simulink model "ModelloParametroNonNoto"  (R2025b)
settings: Solver=ode45  StartTime=0.0  StopTime=20  MaxStep=1e-3  RelTol=1e-3
values from neighbouring files (symbols this model uses):
  a = 5    [main.m]
  K = 2    [main.m]
  ro = 3    [main.m]
settings Model: Creator=Armando  LastModifiedBy=arman

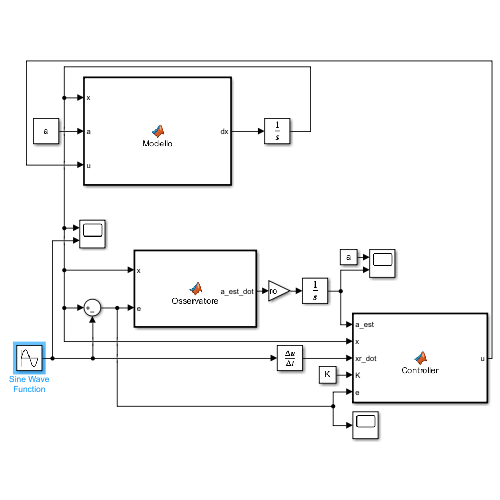
[thumbnail: Simulink's stored preview of the top-level diagram]
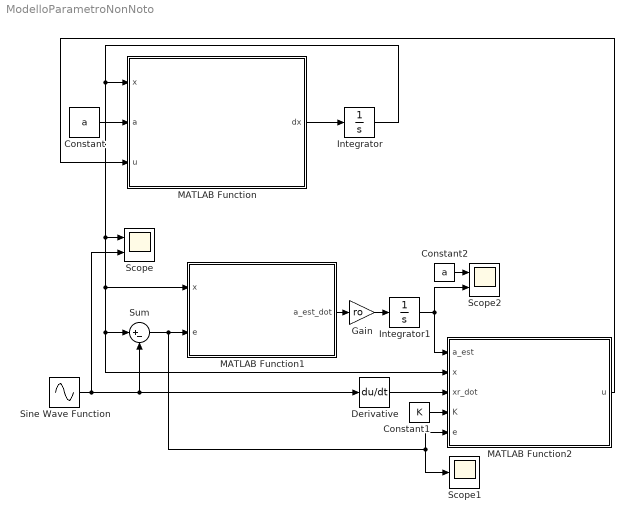
== system ModelloParametroNonNoto ==
  Constant : Constant  Value=a
  Constant1 : Constant  Value=K
  Constant2 : Constant  Value=a
  Derivative : Derivative
  Gain : Gain  Gain=ro
  Integrator : Integrator  InitialCondition=2
  Integrator1 : Integrator  InitialCondition=2
  MATLAB Function : MATLAB Function  TreatAsAtomicUnit=on
  MATLAB Function1 : MATLAB Function  TreatAsAtomicUnit=on
  MATLAB Function2 : MATLAB Function  TreatAsAtomicUnit=on
  Scope : Scope  NumInputPorts=2
      settings: ActiveDisplayYMinimum=-1.3985827995007  ActiveDisplayYMaximum=2.5872376032860807
  Scope1 : Scope
      settings: ActiveDisplayYMinimum=-0.73409681599114474  ActiveDisplayYMaximum=2.40152453242258
  Scope2 : Scope  NumInputPorts=2
      settings: ActiveDisplayYMinimum=1.3806639961716436  ActiveDisplayYMaximum=7.574024034455209  DataLoggingVariableName=ScopeData2
  Sine Wave Function : Sin  SampleTime=0
  Sum : Sum  Inputs=|+-
  wires:
  MATLAB Function/1(dx) -> Integrator/1
  Integrator/1 -> MATLAB Function1/1(x), Sum/1, MATLAB Function2/2(x), Scope/1, MATLAB Function/1(x)
  Constant/1 -> MATLAB Function/2(a)
  Sine Wave Function/1 -> Scope/2, Sum/2, Derivative/1
  Sum/1 -> MATLAB Function1/2(e), Scope1/1, MATLAB Function2/5(e)
  MATLAB Function1/1(a_est_dot) -> Gain/1
  Derivative/1 -> MATLAB Function2/3(xr_dot)
  Constant1/1 -> MATLAB Function2/4(K)
  MATLAB Function2/1(u) -> MATLAB Function/3(u)
  Integrator1/1 -> Scope2/2, MATLAB Function2/1(a_est)
  Gain/1 -> Integrator1/1
  Constant2/1 -> Scope2/1

== matlab function ModelloParametroNonNoto/MATLAB Function1 ==
  data: x input; a_est_dot output; e input
function a_est_dot = Osservatore(x,e)
a_est_dot = x * e;

== matlab function ModelloParametroNonNoto/MATLAB Function ==
  data: x input; a input; u input; dx output
function dx = Modello(x,a,u)
dx = a*x + u;

== matlab function ModelloParametroNonNoto/MATLAB Function2 ==
  data: a_est input; u output; x input; xr_dot input; K input; e input
function u = Controller(a_est,x,xr_dot,K,e)
u = - (a_est * x) + xr_dot - (K*e);
